simulink model "H_Estimation"  (R2025a)
settings: Solver=VariableStepAuto  StartTime=0.0  StopTime=200  FixedStep=1/5120  RelTol=1e-3
values from neighbouring files (symbols this model uses):
  A = [zeros(Dimension), eye(Dimension) ... (first row only)    [spaceABCD.m]    (also in spaceABCD.mat = [0 0 0 0 0 0 0 0 0 0 62247306.1025 -3160223836.01 ... (400 e)
  B = [zeros(Dimension, 2) ... (first row only)    [spaceABCD.m]    (also in spaceABCD.mat = [0 0 0 0 0 0 0 0 0 0 0.522283068671 -34.8509687825 ... (40 e)
  C = zeros(2, 2*Dimension)    [spaceABCD.m]    (also in spaceABCD.mat = [0 0 0 0 0 0 0 0 0 0 0 0 ... (40 elements, 2x20)])
  D = zeros(2, 2)    [spaceABCD.m]    (also in spaceABCD.mat = [0  0; 0  0])
libraries: simulink x2
settings Model: Creator=Administrator  LastModifiedBy=Administrator

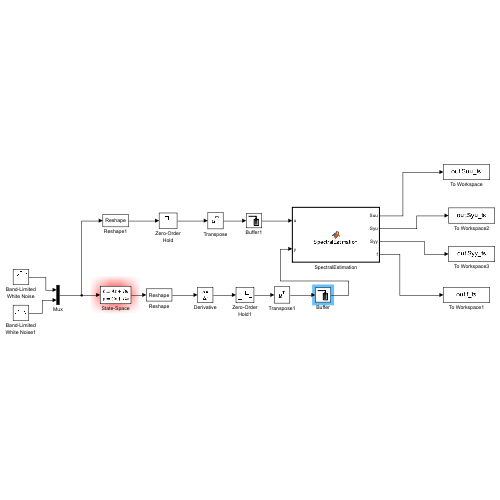
[thumbnail: Simulink's stored preview of the top-level diagram]
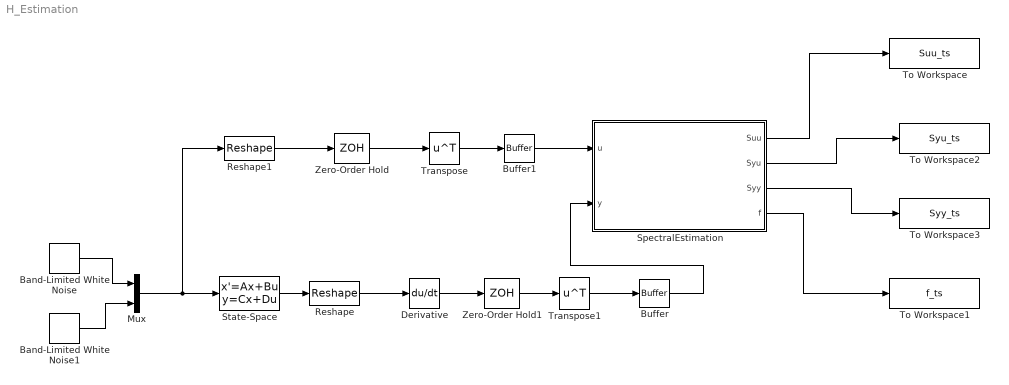
== system H_Estimation ==
  Band-Limited White Noise : simulink/Sources/Band-Limited White Noise  Cov=500  Ts=1/5120  seed=[456]
  Band-Limited White Noise1 : simulink/Sources/Band-Limited White Noise  Cov=500  Ts=1/5120  seed=[123]
  Buffer : Buffer  N=5120  V=2560  OutputFrames=off
  Buffer1 : Buffer  N=5120  V=2560  OutputFrames=off
  Derivative : Derivative
  Mux : Mux  Inputs=2
  Reshape : Reshape  OutputDimensionality=Customize  OutputDimensions=[2,1]
  Reshape1 : Reshape  OutputDimensionality=Customize  OutputDimensions=[2,1]
  SpectralEstimation : MATLAB Function  TreatAsAtomicUnit=on
  State-Space : StateSpace  A=A  B=B  C=C  D=D  InitialCondition=0
  To Workspace : ToWorkspace  VariableName=Suu_ts  SaveFormat=Timeseries  SampleTime=-1
      settings: Save2DSignal=2-D array (concatenate along first dimension)
  To Workspace1 : ToWorkspace  VariableName=f_ts  SaveFormat=Timeseries  SampleTime=-1
      settings: Save2DSignal=2-D array (concatenate along first dimension)
  To Workspace2 : ToWorkspace  VariableName=Syu_ts  SaveFormat=Timeseries  SampleTime=-1
      settings: Save2DSignal=2-D array (concatenate along first dimension)
  To Workspace3 : ToWorkspace  VariableName=Syy_ts  SaveFormat=Timeseries  SampleTime=-1
      settings: Save2DSignal=2-D array (concatenate along first dimension)
  Transpose : Math  Operator=transpose
  Transpose1 : Math  Operator=transpose
  Zero-Order Hold : ZeroOrderHold  SampleTime=1/5120
  Zero-Order Hold1 : ZeroOrderHold  SampleTime=1/5120
  wires:
  Mux/1 -> Reshape1/1, State-Space/1
  Transpose/1 -> Buffer1/1
  Zero-Order Hold1/1 -> Transpose1/1
  Reshape1/1 -> Zero-Order Hold/1
  Buffer/1 -> SpectralEstimation/2(y)
  State-Space/1 -> Reshape/1
  Reshape/1 -> Derivative/1
  SpectralEstimation/4(f) -> To Workspace1/1
  Zero-Order Hold/1 -> Transpose/1
  Band-Limited White Noise/1 -> Mux/1
  Band-Limited White Noise1/1 -> Mux/2
  Transpose1/1 -> Buffer/1
  SpectralEstimation/2(Syu) -> To Workspace2/1
  Buffer1/1 -> SpectralEstimation/1(u)
  SpectralEstimation/1(Suu) -> To Workspace/1
  Derivative/1 -> Zero-Order Hold1/1
  SpectralEstimation/3(Syy) -> To Workspace3/1

== matlab function H_Estimation/SpectralEstimation ==
  data: u input; y input; Suu output; Syu output; Syy output; f output
function [Suu, Syu, Syy, f] = SpectralEstimation(u, y)
% SpectralEstimation 计算MIMO系统的瞬时自功率谱和互功率谱
% 配置：1Hz分辨率 (N=5120, N_half=2561)
% 
% 输入:
%   u: 激励力信号 [5120 x 2] (时域)
%   y: 加速度响应信号 [5120 x 2] (时域)
%
% 输出:
%   Suu: 激励力的自功率谱矩阵 [2561 x 2 x 2] (频域)
%   Syu: 响应与激励的互功率谱矩阵 [2561 x 2 x 2] (频域)
%   f:   频率向量 [2561 x 1]

    % %% 1. 参数定义
    Fs = 5120;          % 采样频率 (Hz)
    N = 5120;           % FFT点数 (1Hz分辨率)
    N_half = N/2 + 1;   % 单边谱的谱线数 (2561)
    
    % %% 2. 加窗 (Hanning Window)
    % 构造汉宁窗 (1024 x 1)
    % 使用 coder.const 优化代码生成，因为窗函数是常数
    %w = 0.5 * (1 - cos(2 * pi * (0:N-1)' / (N-1)));
    % 修改后 (周期性Hann窗)
    w = 0.5 * (1 - cos(2 * pi * (0:N-1)' / N));
    
    % 计算能量恢复系数 (Energy Correction Factor for PSD)
    % 对于 PSD 估计，需要除以窗函数平方和
    W_factor = sum(w.^2); 
    
    % 对输入数据加窗 (Element-wise multiplication)
    % u 和 y 的每一列都会乘以窗函数 w
    u_win = u .* w;
    y_win = y .* w;
    
    % %% 3. FFT 计算
    % 计算 FFT (结果为复数)
    U_fft = fft(u_win);
    Y_fft = fft(y_win);
    
    % 截取单边谱 (1 到 N/2+1)
    U_half = U_fft(1:N_half, :);
    Y_half = Y_fft(1:N_half, :);
    
    % %% 4. 计算功率谱 (PSD) 和 互功率谱 (CPSD)
    % PSD 缩放因子:
    % 2: 因为是单边谱，需要把负频率能量加过来 (DC和Nyquist除外)
    % 1/(Fs * W_factor): PSD的标准归一化
    scale_factor = 2 / (Fs * W_factor);
    
    % 初始化输出矩阵
    % 维度说明: [频率点 x 输出通道 x 输入通道]
    % 这是一个 3D 矩阵，方便后续 system_model.m 提取
    Suu = complex(zeros(N_half, 2, 2));
    Syu = complex(zeros(N_half, 2, 2));
    Syy = complex(zeros(N_half, 2, 2));
    % 循环计算每个频点的谱矩阵
    for k = 1:N_half
        % 提取当前频率 k 的向量 (转置为 2x1 列向量)
        Uk = U_half(k, :).'; 
        Yk = Y_half(k, :).';
        
        % 计算外积 (Outer Product) 生成 2x2 矩阵
        % Suu(k) = Uk * Uk' (共轭转置)
        % Syu(k) = Yk * Uk'
        Suu(k, :, :) = (Uk * Uk') * scale_factor;
        Syu(k, :, :) = (Yk * Uk') * scale_factor;
        % 计算 Syy = Yk * Yk^H
        Syy(k, :, :) = (Yk * Yk') * scale_factor; 
    end
    
    % %% 5. 修正 DC (0Hz) 和 Nyquist 频率分量的缩放
    % 直流分量和奈奎斯特分量不乘 2，所以除回去
    Suu(1, :, :)     = Suu(1, :, :) / 2;
    Suu(end, :, :)   = Suu(end, :, :) / 2;
    Syu(1, :, :)     = Syu(1, :, :) / 2;
    Syu(end, :, :)   = Syu(end, :, :) / 2;
    Syy(1, :, :)   = Syy(1, :, :) / 2;
    Syy(end, :, :) = Syy(end, :, :) / 2;
    
    % %% 6. 生成频率向量
    f = (0:N_half-1)' * (Fs / N);
    
end
